simulink model "LMS_cs"  (R2023a)
settings: Solver=ode5  StartTime=0.0  StopTime=inf  FixedStep=1/200  RelTol=1e-3
PreLoadFcn:
  | mbxruntime.callbacks.PreLoadFcn(bdroot);
PostLoadFcn:
  | mbxruntime.callbacks.PostLoadFcn(bdroot);
InitFcn:
  | mbxruntime.callbacks.InitFcn(bdroot);
StartFcn:
  | mbxruntime.callbacks.StartFcn(bdroot);
StopFcn:
  | mbxruntime.callbacks.StopFcn(bdroot);
model workspace (MAT data in the model file):
  mbox_table : object (value not decoded)
  model_closed = 0
  sim_status = 0
undefined symbols (not defined in the file or in its folder): DiscIntNeverNeededParam, WheelL0, WheelL1, WheelR0, WheelR1
libraries: simulink x462, simulink_extras x117, PreScanSimulinkLibrary x33, PreScanUsefulBlocks x6, instrumentseriallib x5, simulink_need_slupdate x1
(part 7 of 68)

== system LMS_cs/WheelR1_BMW_X5_SUV_9 ==
  WheelR1_BMW_X5_SUV_9 : Inport  Tag=inport/JointActuator  OutDataTypeStr=Bus: PRESCAN_POSE_DATA  SampleTime=2/200  BusOutputAsStruct=on
  Actuator : Subsystem  Tag=VisuJoint  mask(PreScan Sink Block: VisuJoint){UniqueID=3670, Translate_ObjectID3D=BMW_X5_SUV_9.WheelR1, Rotate_ObjectID3D=BMW_X5_SUV_9.WheelR1, TimeStep=2/200, DisplayName=[]}
      mask prompts: UniqueID "Parent Unique ID"; Translate_ObjectID3D "Translate Object Name"; Rotate_ObjectID3D "Rotate Object Name"; TimeStep "Simulation Step"; DisplayName "Display Name"
      mask help:
      | The VisuJoint block provides a way to adapt the location and orientation of a part of an object.
      |
      | For more information, please click Help.
      settings: DeleteFcn=PreScanBlockDeleteFcn;
      mask Help: eval('openHelp(223)')
      mask Display: image(imread('Joint.png'))
  wires:
  WheelR1_BMW_X5_SUV_9/1 -> Actuator/1(Joint)

== system LMS_cs/Audi_A8_Sedan_1/BLR_Demux ==
  Radar : Inport
  Bus Selector1 : BusSelector  OutputSignals=ActiveBeamID[-],Range[m],DopplerVelocity[ms-1],DopplerVelocityX[ms-1],DopplerVelocityY[ms-1],DopplerVelocityZ[ms-1],Theta[deg],Phi[deg],TargetID[-],TargetTypeID[-],EnergyLoss[dB],Alpha[deg],Beta[deg]  OutputAsBus=on
  ScannerSensorLegacyBusConversion : PreScanUsefulBlocks/ScannerSensorLegacyBusConversion  MAXMESSAGES=MAXMESSAGES
  Radar Data : Outport
  wires:
  Bus Selector1/1 -> Radar Data/1
  ScannerSensorLegacyBusConversion/1 -> Bus Selector1/1
  Radar/1 -> ScannerSensorLegacyBusConversion/1

== system LMS_cs/Audi_A8_Sedan_1/BRR_Demux ==
  Radar : Inport
  Bus Selector1 : BusSelector  OutputSignals=ActiveBeamID[-],Range[m],DopplerVelocity[ms-1],DopplerVelocityX[ms-1],DopplerVelocityY[ms-1],DopplerVelocityZ[ms-1],Theta[deg],Phi[deg],TargetID[-],TargetTypeID[-],EnergyLoss[dB],Alpha[deg],Beta[deg]  OutputAsBus=on
  ScannerSensorLegacyBusConversion : PreScanUsefulBlocks/ScannerSensorLegacyBusConversion  MAXMESSAGES=MAXMESSAGES
  Radar Data : Outport
  wires:
  Bus Selector1/1 -> Radar Data/1
  ScannerSensorLegacyBusConversion/1 -> Bus Selector1/1
  Radar/1 -> ScannerSensorLegacyBusConversion/1

== system LMS_cs/Audi_A8_Sedan_1/Dynamics_Simple_3D ==
  DeltaSteer_[deg] : Inport
  Throttle : Inport  Port=2
  Brake : Inport  Port=3
  Initial_Vx_[ms-1] : Inport  Port=4
  AutoManual_OnOff : Inport  Port=5
  Auto_GearShift : Inport  Port=6
  Manual_GearShift : Inport  Port=7
  TyreInfo_in : Inport  Port=8
  Bus Creator : BusCreator  Inputs=14
  Bus Selector : BusSelector  OutputSignals=z_wheelFL_[m],z_wheelFR_[m],z_wheelRL_[m],z_wheelRR_[m]
  Chassis : Subsystem
      mask Display: image(imread('Chassis.png'));
  Engine : Subsystem
      mask Display: image(imread('Engine.png'));
  Gain : Gain  Gain=3.6
  Gear: Auto Manual : Subsystem
  Mux : Mux  Inputs=3
  Radians to Degrees : simulink_extras/Transformations/Radians to Degrees
  Radians to Degrees1 : simulink_extras/Transformations/Radians to Degrees
  Selector : Selector  InputPortWidth=9  IndexOptions=Index vector (dialog)  Indices=7  OutputSizes=1
  Selector1 : Selector  InputPortWidth=9  IndexOptions=Index vector (dialog)  Indices=8  OutputSizes=1
  ShiftLogic : Subsystem
      mask Display: image(imread('Gearshift.png'));
  Transmission : Subsystem
      mask Display: image(imread('Transmission.png'));
  State : Outport
  Vx [m s-1] : Outport  Port=2
  Perf_Params : Outport  Port=3
  z_wheelFL_[m] : Outport  Port=4
  z_wheelFR_[m] : Outport  Port=5
  z_wheelRL_[m] : Outport  Port=6
  z_wheelRR_[m] : Outport  Port=7
  ContactParams : Outport  Port=8
  wires:
  [ax] -> Bus Creator/4  "Ax_[ms-2]"
  [vx] -> Gain/1
  Selector1/1 -> Radians to Degrees1/1
  Selector/1 -> Radians to Degrees/1
  [PD] -> Bus Creator/10  "PDrive_[kW]"
  Radians to Degrees1/1 -> Bus Creator/12  "Pitch_[deg]"
  Radians to Degrees/1 -> Bus Creator/11  "Roll_[deg]"
  [PE] -> Bus Creator/9  "PEngine_[kW]"
  Bus Creator/1 -> Perf_Params/1
  Engine/2(PEngine_[kW]) -> [PE]
  [brake] -> Bus Creator/8  "Brake_[bar]"
  [throttle] -> Bus Creator/7  "Throttle_[perc]"
  [auto_manual] -> Bus Creator/6  "Auto_Manual_[-]"
  [ay] -> Bus Creator/5  "Ay_[ms-2]"
  [gear] -> Bus Creator/3  "Gear_[-]"
  [RPM] -> Bus Creator/2  "NEngine_[rpm]"
  Gain/1 -> Bus Creator/1  "Vx_[kmh-1]"
  Transmission/1(ImpellerTorque_[Nm]) -> Engine/1(ImpellerTorque_[Nm])  "ImpellerTorque_[Nm]"
  Transmission/2(TransmissionTorque_[Nm]) -> Chassis/1(TransmissionTorque_[Nm])  "TransmissionTorque_[Nm]"
  ShiftLogic/1(GearNr) -> ShiftLogic/2(GearNr_[-]), Gear: Auto Manual/3(Auto_Gear)  "GearNr_[-]"
  Engine/1(nEngine_[rpm]) -> Transmission/1(nEngine_[rpm]), [RPM]  "nEngine_[rpm]"
  Chassis/1(State) -> Selector1/1, Selector/1, State/1, Mux/1
  DeltaSteer_[deg]/1 -> Chassis/3(DeltaSteer_[deg])
  Initial_Vx_[ms-1]/1 -> Chassis/4(Initial_Vx_[ms-1])
  Throttle/1 -> [throttle], ShiftLogic/1(Throttle_[%]), Engine/2(Throttle_[%])
  Auto_GearShift/1 -> ShiftLogic/3(Auto_GearShift)
  Chassis/7(TransmissionOut_[rpm]) -> Transmission/3(n_TransmissionOut_[rpm])  "n_driveline_[rpm]"
  Chassis/2(VehicleSpeed_[ms-1]) -> [vx], Vx [m s-1]/1, Mux/2  "vx_[ms-1]"
  AutoManual_OnOff/1 -> [auto_manual], Gear: Auto Manual/1(Auto_Manual)
  Manual_GearShift/1 -> Gear: Auto Manual/2(Manual_Gear)
  Gear: Auto Manual/1(Gear) -> [gear], Transmission/2(GearNr_[-])  "gear"
  [vx] -> ShiftLogic/4(VehSpeed_[ms-1])
  TyreInfo_in/1 -> Chassis/5(TyreInfo_in)
  Brake/1 -> Chassis/2(BrakePressure_[bar]), [brake]
  Chassis/6(PDrive_[kW]) -> [PD]
  Chassis/5(ay_[ms-2]) -> [ay]
  Chassis/4(ax_[ms-2]) -> [ax]
  Chassis/3(Vy_[ms-1]) -> [vy]
  [vx] -> Bus Creator/13  "vx_[ms-1]"
  [vy] -> Bus Creator/14  "vy_[ms-1]"
  Chassis/8(z_wheel_[m]) -> Bus Selector/1, Mux/3  "z_wheel_[m]"
  Bus Selector/1 -> z_wheelFL_[m]/1  "<z_wheelFL_[m]>"
  Bus Selector/2 -> z_wheelFR_[m]/1  "<z_wheelFR_[m]>"
  Bus Selector/3 -> z_wheelRL_[m]/1  "<z_wheelRL_[m]>"
  Bus Selector/4 -> z_wheelRR_[m]/1  "<z_wheelRR_[m]>"
  Mux/1 -> ContactParams/1

== system LMS_cs/Audi_A8_Sedan_1/FLR_Demux ==
  Radar : Inport
  Bus Selector1 : BusSelector  OutputSignals=ActiveBeamID[-],Range[m],DopplerVelocity[ms-1],DopplerVelocityX[ms-1],DopplerVelocityY[ms-1],DopplerVelocityZ[ms-1],Theta[deg],Phi[deg],TargetID[-],TargetTypeID[-],EnergyLoss[dB],Alpha[deg],Beta[deg]  OutputAsBus=on
  ScannerSensorLegacyBusConversion : PreScanUsefulBlocks/ScannerSensorLegacyBusConversion  MAXMESSAGES=MAXMESSAGES
  Radar Data : Outport
  wires:
  Bus Selector1/1 -> Radar Data/1
  ScannerSensorLegacyBusConversion/1 -> Bus Selector1/1
  Radar/1 -> ScannerSensorLegacyBusConversion/1

== system LMS_cs/Audi_A8_Sedan_1/FRR_Demux ==
  Radar : Inport
  Bus Selector1 : BusSelector  OutputSignals=ActiveBeamID[-],Range[m],DopplerVelocity[ms-1],DopplerVelocityX[ms-1],DopplerVelocityY[ms-1],DopplerVelocityZ[ms-1],Theta[deg],Phi[deg],TargetID[-],TargetTypeID[-],EnergyLoss[dB],Alpha[deg],Beta[deg]  OutputAsBus=on
  ScannerSensorLegacyBusConversion : PreScanUsefulBlocks/ScannerSensorLegacyBusConversion  MAXMESSAGES=MAXMESSAGES
  Radar Data : Outport
  wires:
  Bus Selector1/1 -> Radar Data/1
  ScannerSensorLegacyBusConversion/1 -> Bus Selector1/1
  Radar/1 -> ScannerSensorLegacyBusConversion/1

== system LMS_cs/Audi_A8_Sedan_1/JointGroup_WheelDisplacement_V2R ==
  Velocity [m/s] : Inport  SampleTime=TimeStep
  Discrete-Time Integrator : DiscreteIntegrator  SampleTime=TimeStep  ICPrevOutput=DiscIntNeverNeededParam  ICPrevScaledInput=DiscIntNeverNeededParam
  omega=V/Rwheel : Gain  Gain=1/TireRadius
  Rotation [rad] : Outport
  wires:
  Discrete-Time Integrator/1 -> Rotation [rad]/1  "roty"
  omega=V/Rwheel/1 -> Discrete-Time Integrator/1  "rotational speed [rad/s]"
  Velocity [m/s]/1 -> omega=V/Rwheel/1

== system LMS_cs/Audi_A8_Sedan_1/LRR_Demux ==
  Radar : Inport
  Bus Selector1 : BusSelector  OutputSignals=ActiveBeamID[-],Range[m],DopplerVelocity[ms-1],DopplerVelocityX[ms-1],DopplerVelocityY[ms-1],DopplerVelocityZ[ms-1],Theta[deg],Phi[deg],TargetID[-],TargetTypeID[-],EnergyLoss[dB],Alpha[deg],Beta[deg]  OutputAsBus=on
  ScannerSensorLegacyBusConversion : PreScanUsefulBlocks/ScannerSensorLegacyBusConversion  MAXMESSAGES=MAXMESSAGES
  Radar Data : Outport
  wires:
  Bus Selector1/1 -> Radar Data/1
  ScannerSensorLegacyBusConversion/1 -> Bus Selector1/1
  Radar/1 -> ScannerSensorLegacyBusConversion/1

== system LMS_cs/Audi_A8_Sedan_1/Lane Keeping Algorithm ==
  Sensor Data : Inport
  Add : Sum
  Add1 : Sum
  Add2 : Sum
  Bus Selector : BusSelector  OutputSignals=ScanAtSensor.SliceCenterCoordsX,ScanAtSensor.SliceCenterCoordsY,ScanAtDistance1.SliceCenterCoordsX,ScanAtDistance1.SliceCenterCoordsY,ScanAtSensor.RightLaneIntersection1.WorldCoordinateX,ScanAtSensor.RightLaneIntersection1.WorldCoordinateY,ScanAtDistance1.RightLaneIntersection1.WorldCoordinateX,ScanAtDistance1.RightLaneIntersection1.WorldCoordinateY
  Bus Selector1 : BusSelector  OutputSignals=ScanAtDistance1.LeftLaneIntersection1.DistanceFromScanCenter,ScanAtDistance1.RightLaneIntersection1.DistanceFromScanCenter,ScanAtDistance1.RoadIdUnderSliceCenter
  Constant : Constant  Value=-0.5
  Display{,1..18} (19 alike) : Display
  Divide : Product  Inputs=/*
  Scaler1 : Constant  Value=1250
  Scaler2 : Gain  Gain=-250
  Steering 0 : Constant  Value=0
  Switch : Switch  Criteria=u2 > Threshold  SaturateOnIntegerOverflow=off  InputSameDT=off
  "angular error " : M-S-Function  FunctionName=angular_error_msfun
      mask Display:
      | port_label('input',1,'cx1')
      | port_label('input',2,'cy1')
      | port_label('input',3,'cx2')
      | port_label('input',4,'cy2')
      | port_label('input',5,'lsx1')
      | port_label('input',6,'lsy1')
      | port_label('input',7,'lsx2')
      | port_label('input',8,'lsy2')
      | port_label('input',9,'scaler')
      | port_label('output',1,'angle')
  Steering Angle : Outport
  wires:
  Switch/1 -> Steering Angle/1
  Steering 0/1 -> Switch/3
  Bus Selector1/3 -> Display2/1, Switch/2  "<RoadIdUnderSliceCenter>"
  Add2/1 -> Display1/1, Switch/1
  Sensor Data/1 -> Bus Selector1/1, Bus Selector/1
  Bus Selector1/1 -> Display12/1, Display4/1, Add/1  "<DistanceFromScanCenter>"
  Bus Selector1/2 -> Display13/1, Divide/2, Add/2  "<DistanceFromScanCenter>"
  Add/1 -> Display14/1, Divide/1
  Divide/1 -> Display16/1, Display15/1, Add1/2
  Constant/1 -> Add1/1
  Add1/1 -> Display17/1, Scaler2/1
  Scaler2/1 -> Display18/1, Add2/2
  Bus Selector/1 -> Display3/1, "angular error "/1  "<SliceCenterCoordsX>"
  Bus Selector/2 -> Display5/1, "angular error "/2  "<SliceCenterCoordsY>"
  Bus Selector/3 -> Display6/1, "angular error "/3  "<SliceCenterCoordsX>"
  Bus Selector/4 -> "angular error "/4, Display7/1  "<SliceCenterCoordsY>"
  Bus Selector/5 -> Display8/1, "angular error "/5  "<WorldCoordinateX>"
  Bus Selector/6 -> Display9/1, "angular error "/6  "<WorldCoordinateY>"
  Bus Selector/7 -> Display10/1, "angular error "/7  "<WorldCoordinateX>"
  Bus Selector/8 -> Display11/1, "angular error "/8  "<WorldCoordinateY>"
  "angular error "/1 -> Display/1, Add2/1
  Scaler1/1 -> "angular error "/9

== system LMS_cs/Audi_A8_Sedan_1/LaneMarkerSensor_1_Data ==
  In1 : Inport
  Bus Creator : BusCreator  Inputs='SliceCount','ScanAtSensor','ScanAtDistance1','ScanAtDistance2','ScanAtDistance3'
  Constant : Constant
  Constant1 : Constant  Value=NUMBEROFSLICES
  Constant2 : Constant  Value=2
  Constant3 : Constant  Value=3
  Constant4 : Constant  Value=4
  Data Type Conversion : DataTypeConversion  OutDataTypeStr=int32  SaturateOnIntegerOverflow=off  RndMeth=Floor
  If{,1..3} (4 alike) : If  NumInputs=2  IfExpression=u1 >= u2  ShowElse=off
  If Action Subsystem1 : Subsystem  TreatAsAtomicUnit=on
  If Action Subsystem2 : Subsystem  TreatAsAtomicUnit=on
  If Action Subsystem3 : Subsystem  TreatAsAtomicUnit=on
  If Action Subsystem4 : Subsystem  TreatAsAtomicUnit=on
  Merge{,1..3} (4 alike) : Merge  InitialOutput=0
  Zero-filled data bus{,1..3} (4 alike) : Constant  Value=0  VectorParams1D=off  OutDataTypeStr=Bus: PRESCAN_LANEMARKER_DATA  SampleTime=TimeStep
  Detection Data : Outport
  wires:
  Data Type Conversion/1 -> Bus Creator/1  "SliceCount"
  In1/1 -> If Action Subsystem2/1(In1), If Action Subsystem4/1(In1), If Action Subsystem3/1(In1), If Action Subsystem1/1(In1)
  Zero-filled data bus3/1 -> Merge3/1
  Zero-filled data bus2/1 -> Merge2/1
  Zero-filled data bus1/1 -> Merge1/1
  Zero-filled data bus/1 -> Merge/1
  Merge3/1 -> Bus Creator/5  "ScanAtDistance3"
  Merge2/1 -> Bus Creator/4  "ScanAtDistance2"
  Merge1/1 -> Bus Creator/3  "ScanAtDistance1"
  If3/1 -> If Action Subsystem4/Action
  If Action Subsystem4/1(Out1) -> Merge3/2
  Constant4/1 -> If3/2, If Action Subsystem4/2(In2)
  If2/1 -> If Action Subsystem3/Action
  If Action Subsystem3/1(Out1) -> Merge2/2
  Constant3/1 -> If Action Subsystem3/2(In2), If2/2
  If1/1 -> If Action Subsystem1/Action
  If Action Subsystem1/1(Out1) -> Merge1/2
  Constant2/1 -> If Action Subsystem1/2(In2), If1/2
  Merge/1 -> Bus Creator/2  "ScanAtSensor"
  Bus Creator/1 -> Detection Data/1
  If/1 -> If Action Subsystem2/Action
  If Action Subsystem2/1(Out1) -> Merge/2
  Constant/1 -> If Action Subsystem2/2(In2), If/2
  Constant1/1 -> Data Type Conversion/1, If3/1, If2/1, If1/1, If/1

== system LMS_cs/Audi_A8_Sedan_1/PathFollower_1 ==
  TrajOffset_x,y,Y [m,m,deg] : Inport
  ActorOffset_Left(+) / Right(-) [m] : Inport  Port=2
  position x,y,Y [m,m,deg] : Inport  Port=3
  Initial Velocity [m/s] : Inport  Port=4
  Desired Velocity [m/s] : Inport  Port=5
  velocity [m/s] : Inport  Port=6
  CTRL REFERENCES : Subsystem
  Calculate shifted p0 wrt COG : Subsystem
  DELTA CTRL : Subsystem
  Demux : Demux  Outputs=3
  Gain : Gain  Gain=1*pi/180
  Goto Tag Visibility : GotoTagVisibility  GotoTag=PreviewDistance
  Goto Tag Visibility1 : GotoTagVisibility  GotoTag=v_actual
  Memory1 : Memory
  Memory2 : Memory
  Memory3 : Memory
  Mux : Mux  Inputs=3
  Preview distance velocity dependent : Lookup  InputValues=[0 20 30 40 50 60 70 80 90 100 120]  Table=[1 1 2 3 4 5 6 7 10 13.33 20]  SaturateOnIntegerOverflow=off
  THROTTLE CTRL : Subsystem
  sign1 : Gain  Gain=3.6
  delta_steerwheel [deg] : Outport
  throttle [%] : Outport  Port=2
  brake pressure [bar] : Outport  Port=3
  v0 [m/s] : Outport  Port=4
  Auto_GearShift : Outport  Port=5
  Actor/Traj_distance [m] : Outport  Port=6
  Actor/Traj_angle [deg] : Outport  Port=7
  tag scope: PreviewDistance=scoped, v_actual=scoped
  wires:
  Memory3/1 -> CTRL REFERENCES/4(ActorOffset_Left(+) / Right(-)_[m])
  THROTTLE CTRL/4(Auto_GearShift) -> Auto_GearShift/1
  THROTTLE CTRL/2(brake pressure [bar]) -> brake pressure [bar]/1
  Memory2/1 -> THROTTLE CTRL/1(v_actual [m/s]), [v_actual]
  Memory1/1 -> DELTA CTRL/1(p0), CTRL REFERENCES/1(Pos x,y,Y [m,m,rad])
  sign1/1 -> Preview distance velocity dependent/1
  Initial Velocity [m/s]/1 -> THROTTLE CTRL/3(Initial Velocity [m/s])
  velocity [m/s]/1 -> Memory2/1
  CTRL REFERENCES/1(pvp  [m,m]) -> DELTA CTRL/2(pvp)
  CTRL REFERENCES/2(pref_pvp [m,m]) -> DELTA CTRL/3(pref_pvp)
  Gain/1 -> Mux/3
  DELTA CTRL/1(delta_steerwheel [deg]) -> delta_steerwheel [deg]/1
  Mux/1 -> CTRL REFERENCES/3(TrajOffset [m,m,rad])
  CTRL REFERENCES/3(pref_0 [m,m]) -> DELTA CTRL/4(pref0)
  THROTTLE CTRL/3(v0 [m/s]) -> v0 [m/s]/1
  THROTTLE CTRL/1(throttle [%]) -> throttle [%]/1
  [v_actual] -> sign1/1
  Preview distance velocity dependent/1 -> [PreviewDistance], CTRL REFERENCES/2(Position Preview Distance [m])
  Desired Velocity [m/s]/1 -> THROTTLE CTRL/2(Desired Velocity [m/s])
  ActorOffset_Left(+) / Right(-) [m]/1 -> Memory3/1
  Demux/1 -> Mux/1
  Demux/2 -> Mux/2
  Demux/3 -> Gain/1
  TrajOffset_x,y,Y [m,m,deg]/1 -> Demux/1
  Calculate shifted p0 wrt COG/1(position x,y,Y [m,m,rad]) -> Memory1/1
  position x,y,Y [m,m,deg]/1 -> Calculate shifted p0 wrt COG/1(position x,y,Y [m,m,deg])
  CTRL REFERENCES/4(Actor/Traj_distance [m]) -> Actor/Traj_distance [m]/1
  CTRL REFERENCES/5(Actor/Traj_angle [deg]) -> Actor/Traj_angle [deg]/1

== system LMS_cs/Audi_A8_Sedan_1/PreScan_Contact_Sensor ==
  ContactParams : Inport  SampleTime=TimeStep
  Steer Angle Front [deg] : Inport  Port=2
  Steer Angle Rear [deg] : Inport  Port=3
  Bus Creator2 : BusCreator  Inputs=4
  Demux : Demux
  Demux1 : Demux  Outputs=[9 1 4]
  Demux2 : Demux
  For All Wheel Contacts : Subsystem  TreatAsAtomicUnit=on
  Mux6 : Mux  Inputs=2
  Subsystem : Subsystem  mask{NumberOfWheels=4, MaxContactPoints=4, WheelRadius=wheelRadius, WheelWidth=0.2}
      mask prompts: NumberOfWheels "Number of Wheels"; MaxContactPoints "Maximum number of Contact Points"; WheelRadius "Wheel Radius"; WheelWidth "Wheel Width"
      mask Display: disp('Contact Sensor')
  Tire Collision Demux : Subsystem
  Tire Collision Demux1 : Subsystem
  Tire Collision Demux2 : Subsystem
  Tire Collision Demux3 : Subsystem
  Vehicle Local to World : Subsystem
  Wheels = 4 : Subsystem  mask{NumberOfWheels=4}
      mask prompts: NumberOfWheels "Number of Wheels"
      mask Display:
      | port_label('input', 1,'Vehicle wrt World')
      | port_label('input', 2,'Wheels wrt World')
  Wheels Local to World : Subsystem  Tag=MuxWheels  mask(PreScan Mux Block:){}
      settings: DeleteFcn=PreScanBlockDeleteFcn;
  Results : Outport
  wires:
  Mux6/1 -> Wheels = 4/1(Vehicle wrt World)
  Wheels = 4/1(WheelPoses) -> Subsystem/1(In1)
  Demux/1 -> Tire Collision Demux/1(demux in)
  Demux/2 -> Tire Collision Demux1/1(demux in)
  Demux/3 -> Tire Collision Demux2/1(demux in)
  Demux/4 -> Tire Collision Demux3/1(demux in)
  Tire Collision Demux/1(bus out) -> Bus Creator2/1  "TireFL"
  Tire Collision Demux1/1(bus out) -> Bus Creator2/2  "TireFR"
  Tire Collision Demux2/1(bus out) -> Bus Creator2/3  "TireRL"
  Tire Collision Demux3/1(bus out) -> Bus Creator2/4  "TireRR"
  Vehicle Local to World/1(Position) -> Mux6/1
  Vehicle Local to World/2(Orientation) -> Mux6/2
  Wheels Local to World/1(Wheel Poses) -> Wheels = 4/2(Wheels wrt World)
  Demux1/2 -> Wheels Local to World/3(Velocity [m/s])
  Demux2/1 -> Wheels Local to World/4(zDisp FL [m])
  Demux2/2 -> Wheels Local to World/5(zDisp FR [m])
  Demux2/3 -> Wheels Local to World/6(zDisp RL [m])
  Demux2/4 -> Wheels Local to World/7(zDisp RR [m])
  Steer Angle Front [deg]/1 -> Wheels Local to World/1(Steer Angle Front [deg])
  Steer Angle Rear [deg]/1 -> Wheels Local to World/2(Steer Angle Rear [deg])
  Bus Creator2/1 -> Results/1
  ContactParams/1 -> Demux1/1
  Demux1/1 -> Vehicle Local to World/1(State)
  Demux1/3 -> Demux2/1
  Subsystem/1(Out1) -> For All Wheel Contacts/1(In1)
  For All Wheel Contacts/1(Out1) -> Demux/1

== system LMS_cs/Audi_A8_Sedan_1/SELF_Demux ==
  SELF : Inport  OutDataTypeStr=Bus: PRESCAN_SELFSENSORDATA
  Bus Selector : BusSelector  OutputSignals=PositionX,PositionY,PositionZ,OrientationRoll,OrientationPitch,OrientationYaw,Velocity,Yaw_rate,Lat,Long,Alt
  Demux2 : Demux  Outputs=3
  Gain : Gain  Gain=180/pi
  Gain1 : Gain  Gain=180/pi
  Vector Concatenate1 : Concatenate  NumInputs=3
  compas converter : Subsystem
  x [m] : Outport
  y [m] : Outport  Port=2
  z [m] : Outport  Port=3
  rotx [deg] : Outport  Port=4
  roty [deg] : Outport  Port=5
  rotz [deg] : Outport  Port=6
  GPS lat [deg] : Outport  Port=7
  GPS long [deg] : Outport  Port=8
  GPS alt [m] : Outport  Port=9
  velocity [m/s] : Outport  Port=10
  heading [deg] : Outport  Port=11
  yaw rate [deg/s] : Outport  Port=12
  wires:
  Bus Selector/11 -> GPS alt [m]/1  "<Alt>"
  Bus Selector/10 -> GPS long [deg]/1  "<Long>"
  Bus Selector/9 -> GPS lat [deg]/1  "<Lat>"
  Bus Selector/8 -> Gain1/1  "<Yaw_rate>"
  Bus Selector/7 -> velocity [m/s]/1  "<Velocity>"
  Bus Selector/6 -> compas converter/1(rotz [rad]), Vector Concatenate1/3  "<OrientationYaw>"
  Bus Selector/5 -> Vector Concatenate1/2  "<OrientationPitch>"
  Bus Selector/4 -> Vector Concatenate1/1  "<OrientationRoll>"
  Vector Concatenate1/1 -> Gain/1
  Bus Selector/3 -> z [m]/1  "<PositionZ>"
  Bus Selector/2 -> y [m]/1  "<PositionY>"
  Bus Selector/1 -> x [m]/1  "<PositionX>"
  SELF/1 -> Bus Selector/1
  Gain/1 -> Demux2/1
  Demux2/1 -> rotx [deg]/1
  Demux2/2 -> roty [deg]/1
  Demux2/3 -> rotz [deg]/1
  compas converter/1(heading [deg]) -> heading [deg]/1
  Gain1/1 -> yaw rate [deg/s]/1

== system LMS_cs/Audi_A8_Sedan_1/SRR_Demux ==
  Radar : Inport
  Bus Selector1 : BusSelector  OutputSignals=ActiveBeamID[-],Range[m],DopplerVelocity[ms-1],DopplerVelocityX[ms-1],DopplerVelocityY[ms-1],DopplerVelocityZ[ms-1],Theta[deg],Phi[deg],TargetID[-],TargetTypeID[-],EnergyLoss[dB],Alpha[deg],Beta[deg]  OutputAsBus=on
  ScannerSensorLegacyBusConversion : PreScanUsefulBlocks/ScannerSensorLegacyBusConversion  MAXMESSAGES=MAXMESSAGES
  Radar Data : Outport
  wires:
  Bus Selector1/1 -> Radar Data/1
  ScannerSensorLegacyBusConversion/1 -> Bus Selector1/1
  Radar/1 -> ScannerSensorLegacyBusConversion/1

== system LMS_cs/Audi_A8_Sedan_1/STATE_Audi_A8_Sedan_1 ==
  State : Inport  SampleTime=TimeStep
  Bus Creator : BusCreator  Inputs=15  OutDataTypeStr=Bus: PRESCAN_STATEACTUATORDATA  NonVirtualBus=on
  Demux : Demux  Outputs=15
  iniBODYAngles wrtVEH [rad] : Constant  Value=[Roll0 Pitch0 0]  SampleTime=TimeStep
  iniVEHAngles wrtGLOB [rad] : Constant  Value=[0 0 Yaw0]  SampleTime=TimeStep
  iniVEHposition wrtGLOB [m] : Constant  Value=[x0 y0 z0]  SampleTime=TimeStep
  state2FullState : PreScanSimulinkLibrary/state2FullState  SystemSampleTime=-1  VariantActivationTime=update diagram  Latency=0  AutoFrameSizeCalculation=off
  StateBus : Outport  OutDataTypeStr=Bus: PRESCAN_STATEACTUATORDATA
  wires:
  Bus Creator/1 -> StateBus/1
  State/1 -> state2FullState/1
  state2FullState/1 -> Demux/1
  iniVEHposition wrtGLOB [m]/1 -> state2FullState/2
  iniBODYAngles wrtVEH [rad]/1 -> state2FullState/3
  iniVEHAngles wrtGLOB [rad]/1 -> state2FullState/4
  Demux/1 -> Bus Creator/1  "PositionX"
  Demux/2 -> Bus Creator/2  "PositionY"
  Demux/3 -> Bus Creator/3  "PositionZ"
  Demux/4 -> Bus Creator/4  "VelocityX"
  Demux/5 -> Bus Creator/5  "VelocityY"
  Demux/6 -> Bus Creator/6  "VelocityZ"
  Demux/7 -> Bus Creator/7  "AccelerationX"
  Demux/8 -> Bus Creator/8  "AccelerationY"
  Demux/9 -> Bus Creator/9  "AccelerationZ"
  Demux/10 -> Bus Creator/10  "OrientationRoll"
  Demux/11 -> Bus Creator/11  "OrientationPitch"
  Demux/12 -> Bus Creator/12  "OrientationYaw"
  Demux/13 -> Bus Creator/13  "AngularVelocityRoll"
  Demux/14 -> Bus Creator/14  "AngularVelocityPitch"
  Demux/15 -> Bus Creator/15  "AngularVelocityYaw"

== system LMS_cs/Audi_A8_Sedan_1/State2PathFollowerCnv ==
  State BUS : Inport  OutDataTypeStr=Bus: PRESCAN_STATEACTUATORDATA
  Bus Selector : BusSelector  OutputSignals=AngularVelocityYaw,VelocityX,VelocityY,PositionX,PositionY,OrientationYaw
  Radians to Degrees : simulink_extras/Transformations/Radians to Degrees
  Radians to Degrees1 : simulink_extras/Transformations/Radians to Degrees
  SELF2PathFollowerMux : Mux  Tag=SELF2PathFollowerMux  Inputs=3
  velocity magnitude : Math  Operator=hypot  SignedPower=on
  Yaw rate [deg/s] : Outport
  velocity [m/s] : Outport  Port=2
  position x,y,Y [m,m,deg] : Outport  Port=3
  wires:
  Radians to Degrees1/1 -> Yaw rate [deg/s]/1
  Bus Selector/1 -> Radians to Degrees1/1  "<AngularVelocityYaw>"
  velocity magnitude/1 -> velocity [m/s]/1
  SELF2PathFollowerMux/1 -> position x,y,Y [m,m,deg]/1
  State BUS/1 -> Bus Selector/1
  Bus Selector/2 -> velocity magnitude/1  "<VelocityX>"
  Bus Selector/3 -> velocity magnitude/2  "<VelocityY>"
  Radians to Degrees/1 -> SELF2PathFollowerMux/3
  Bus Selector/6 -> Radians to Degrees/1  "<OrientationYaw>"
  Bus Selector/4 -> SELF2PathFollowerMux/1  "<PositionX>"
  Bus Selector/5 -> SELF2PathFollowerMux/2  "<PositionY>"

== system LMS_cs/Audi_A8_Sedan_1/Trajectories ==
  Traj2State1 : Subsystem  Tag=Traj2State  mask(PreScan Demux Block:){}
      settings: DeleteFcn=PreScanBlockDeleteFcn;
  TrajCoGOffset : Subsystem  Tag=TrajCoGOffset  mask(Trajectory CoG Offset block){CoGOffsetZ=0.55, InitRoll=0, InitPitch=0}
      mask prompts: CoGOffsetZ "Z-component of CoG Offset [m]:"; InitRoll "Initial Roll angle [deg]:"; InitPitch "Initial Pitch angle [deg]:"
      mask help: A trajectory follows the surface of the road. However the position of a actor is based on the actor's Center of Gravity, which is typically above the road. This block converts from the trajectory along the road surface to the trajectory of the actor's CoG by realigning the z-component of the CoG offset to be normal to the road.
      settings: DeleteFcn=PreScanBlockDeleteFcn;
  Trajectory_1 : Subsystem  Tag=Trajectory  mask(PreScan Source Block: Trajectory){FileName='Trajectory_1.mat', TimeStep=2/200}
      mask prompts: TimeStep "Time Step [s]"
      mask help:
      | The Trajectory block contains the trajectories defined in the PreScan Experiment Editor. The output of the trajectory block is the (vehicle) State.
      |
      | For more information, please click Help.
      mask init:
      | EXPROOT=pwd;  % TODO better construction for locating base experiment
      | 
      | trajfilename = fullfile(EXPROOT,'Trajectories',FileName);
      | load(trajfilename);
      | trajectory=trajectory';
      | 
      | traj.time=trajectory(:,1);%[];
      | traj.signals.values=trajectory(:,2:19);
      | traj.dimensions=18;
      | traj.label='';
      | 
      | SampleTime=traj.time(2)-traj.time(1);
      settings: DeleteFcn=PreScanBlockDeleteFcn;
      mask Help: eval('openHelp(312)')
      mask Display: fprintf(FileName)
  Trajectory_1_Offset : Constant  Tag=TrajectoryOffset  Value="[0  0  0  0  0  0]"
  State : Outport  Tag=TrajOutport
  wires:
  Trajectory_1/1(trajectory) -> Traj2State1/1(Traj Org)
  Trajectory_1_Offset/1 -> Traj2State1/2(Offset)
  TrajCoGOffset/1(State Out) -> State/1
  Traj2State1/1(state) -> TrajCoGOffset/1(State In)

== system LMS_cs/Audi_A8_Sedan_1/WheelDisplacement_Mux ==
  Steering Angle Front [rad] : Inport  Tag=inport/JointGroup  SampleTime=2/200  BusOutputAsStruct=on
  Steering Angle Rear [rad] : Inport  Tag=inport/JointGroup  Port=2  SampleTime=2/200  BusOutputAsStruct=on
  Rotation [rad] : Inport  Tag=inport/JointGroup  Port=3  SampleTime=2/200  BusOutputAsStruct=on
  zDisp FL [m] : Inport  Tag=inport/JointGroup  Port=4  SampleTime=2/200  BusOutputAsStruct=on
  zDisp FR [m] : Inport  Tag=inport/JointGroup  Port=5  SampleTime=2/200  BusOutputAsStruct=on
  zDisp RL [m] : Inport  Tag=inport/JointGroup  Port=6  SampleTime=2/200  BusOutputAsStruct=on
  zDisp RR [m] : Inport  Tag=inport/JointGroup  Port=7  SampleTime=2/200  BusOutputAsStruct=on
  Ground_{1..12} (12 alike) : Ground
  WheelL0_Mux : Subsystem  Tag=mux/Joint  mask(PreScan Mux Block){DisplayName=WheelL0}
      mask prompts: DisplayName "Display Name"
      mask help:
      | This block simulates a generic joint used for generic models. This joint can be enabled/disabled from the GUI.
      |
      | For more information, please click Help.
      settings: DeleteFcn=PreScanBlockDeleteFcn;
      mask Help: eval('openHelp(254)')
  WheelL1_Mux : Subsystem  Tag=mux/Joint  mask(PreScan Mux Block){DisplayName=WheelL1}
      mask prompts: DisplayName "Display Name"
      mask help:
      | This block simulates a generic joint used for generic models. This joint can be enabled/disabled from the GUI.
      |
      | For more information, please click Help.
      settings: DeleteFcn=PreScanBlockDeleteFcn;
      mask Help: eval('openHelp(254)')
  WheelR0_Mux : Subsystem  Tag=mux/Joint  mask(PreScan Mux Block){DisplayName=WheelR0}
      mask prompts: DisplayName "Display Name"
      mask help:
      | This block simulates a generic joint used for generic models. This joint can be enabled/disabled from the GUI.
      |
      | For more information, please click Help.
      settings: DeleteFcn=PreScanBlockDeleteFcn;
      mask Help: eval('openHelp(254)')
  WheelR1_Mux : Subsystem  Tag=mux/Joint  mask(PreScan Mux Block){DisplayName=WheelR1}
      mask prompts: DisplayName "Display Name"
      mask help:
      | This block simulates a generic joint used for generic models. This joint can be enabled/disabled from the GUI.
      |
      | For more information, please click Help.
      settings: DeleteFcn=PreScanBlockDeleteFcn;
      mask Help: eval('openHelp(254)')
  WheelL0_Audi_A8_Sedan_1 : Outport  Tag=outport/JointActuator  OutDataTypeStr=Bus: PRESCAN_POSE_DATA  SampleTime=2/200
  WheelL1_Audi_A8_Sedan_1 : Outport  Tag=outport/JointActuator  Port=2  OutDataTypeStr=Bus: PRESCAN_POSE_DATA  SampleTime=2/200
  WheelR0_Audi_A8_Sedan_1 : Outport  Tag=outport/JointActuator  Port=3  OutDataTypeStr=Bus: PRESCAN_POSE_DATA  SampleTime=2/200
  WheelR1_Audi_A8_Sedan_1 : Outport  Tag=outport/JointActuator  Port=4  OutDataTypeStr=Bus: PRESCAN_POSE_DATA  SampleTime=2/200
  wires:
  WheelL0_Mux/1(Joint) -> WheelL0_Audi_A8_Sedan_1/1
  WheelL1_Mux/1(Joint) -> WheelL1_Audi_A8_Sedan_1/1
  WheelR0_Mux/1(Joint) -> WheelR0_Audi_A8_Sedan_1/1
  WheelR1_Mux/1(Joint) -> WheelR1_Audi_A8_Sedan_1/1
  Steering Angle Front [rad]/1 -> WheelR0_Mux/6(Yaw [rad]), WheelL0_Mux/6(Yaw [rad])
  Steering Angle Rear [rad]/1 -> WheelR1_Mux/6(Yaw [rad]), WheelL1_Mux/6(Yaw [rad])
  Rotation [rad]/1 -> WheelR0_Mux/5(Pitch [rad]), WheelL0_Mux/5(Pitch [rad]), WheelR1_Mux/5(Pitch [rad]), WheelL1_Mux/5(Pitch [rad])
  zDisp FL [m]/1 -> WheelL0_Mux/3(Z [m])
  zDisp FR [m]/1 -> WheelR0_Mux/3(Z [m])
  zDisp RL [m]/1 -> WheelL1_Mux/3(Z [m])
  zDisp RR [m]/1 -> WheelR1_Mux/3(Z [m])
  Ground_1/1 -> WheelL0_Mux/1(X [m])
  Ground_2/1 -> WheelL0_Mux/2(Y [m])
  Ground_3/1 -> WheelL0_Mux/4(Roll [rad])
  Ground_4/1 -> WheelL1_Mux/1(X [m])
  Ground_5/1 -> WheelL1_Mux/2(Y [m])
  Ground_6/1 -> WheelL1_Mux/4(Roll [rad])
  Ground_7/1 -> WheelR0_Mux/1(X [m])
  Ground_8/1 -> WheelR0_Mux/2(Y [m])
  Ground_9/1 -> WheelR0_Mux/4(Roll [rad])
  Ground_10/1 -> WheelR1_Mux/1(X [m])
  Ground_11/1 -> WheelR1_Mux/2(Y [m])
  Ground_12/1 -> WheelR1_Mux/4(Roll [rad])

== system LMS_cs/Audi_A8_Sedan_1/concatinate Frame ==
  " Desired Velocity" : Inport
  Heading : Inport  Port=2
  " LRR_Range" : Inport  Port=3
  LRR_RelativeVelocity : Inport  Port=4
  " SRR_Range" : Inport  Port=5
  " SRR_RelativeVelocity" : Inport  Port=6
  " FLR_Range" : Inport  Port=7
  " FLR_RelativeVelocity" : Inport  Port=8
  FLR_Azimuth : Inport  Port=9
  " FRR_Range" : Inport  Port=10
  " FRR_RelativeVelocity" : Inport  Port=11
  " FRR_Azimuth" : Inport  Port=12
  " BRR_Range" : Inport  Port=13
  " BRR_RelativeVelocity" : Inport  Port=14
  " BRR_Azimuth" : Inport  Port=15
  " BLR_Range" : Inport  Port=16
  " BLR_RelativeVelocity" : Inport  Port=17
  " BLR_Azimuth" : Inport  Port=18
  Velocity : Inport  Port=19
  laneMarkerX_D0 : Inport  Port=20
  laneMarkerY_D0 : Inport  Port=21
  laneMarkerX_D1 : Inport  Port=22
  laneMarkerY_D1 : Inport  Port=23
  worldrX_D0 : Inport  Port=24
  worldY_D0 : Inport  Port=25
  worldX_D1 : Inport  Port=26
  worldY_D1 : Inport  Port=27
  laneMarkerLeft_D1 : Inport  Port=28
  laneMarkerRight_D1 : Inport  Port=29
  roadID : Inport  Port=30
  String Concatenate : StringConcatenate  Inputs=61
  String Constant : StringConstant  String="\"*\""
  String Constant{1..4,6..30} (29 alike) : StringConstant  String="\";\""
  String Constant5 : StringConstant  String="\"#\""
  String to ASCII : StringToASCII  OutputVectorSize=255
  To String{,1..29} (30 alike) : ToString
  Frame : Outport  VectorParamsAs1DForOutWhenUnconnected=off
  wires:
  String to ASCII/1 -> Frame/1
  " SRR_Range"/1 -> To String4/1
  To String4/1 -> String Concatenate/10
  String Constant3/1 -> String Concatenate/7
  Heading/1 -> To String1/1
  To String2/1 -> String Concatenate/6
  String Constant1/1 -> String Concatenate/3
  " Desired Velocity"/1 -> To String/1
  String Constant/1 -> String Concatenate/1
  " LRR_Range"/1 -> To String2/1
  To String1/1 -> String Concatenate/4
  To String3/1 -> String Concatenate/8
  To String/1 -> String Concatenate/2
  LRR_RelativeVelocity/1 -> To String3/1
  String Constant4/1 -> String Concatenate/9
  String Constant2/1 -> String Concatenate/5
  String Concatenate/1 -> String to ASCII/1
  String Constant6/1 -> String Concatenate/11
  String Constant7/1 -> String Concatenate/13
  String Constant8/1 -> String Concatenate/15
  String Constant9/1 -> String Concatenate/17
  String Constant10/1 -> String Concatenate/19
  String Constant11/1 -> String Concatenate/21
  String Constant12/1 -> String Concatenate/23
  String Constant13/1 -> String Concatenate/25
  String Constant14/1 -> String Concatenate/27
  String Constant15/1 -> String Concatenate/29
  String Constant16/1 -> String Concatenate/31
  String Constant17/1 -> String Concatenate/33
  String Constant18/1 -> String Concatenate/35
  " SRR_RelativeVelocity"/1 -> To String5/1
  To String5/1 -> String Concatenate/12
  " FLR_Range"/1 -> To String6/1
  To String6/1 -> String Concatenate/14
  " FLR_RelativeVelocity"/1 -> To String7/1
  To String7/1 -> String Concatenate/16
  FLR_Azimuth/1 -> To String8/1
  To String8/1 -> String Concatenate/18
  " FRR_Range"/1 -> To String9/1
  To String9/1 -> String Concatenate/20
  " FRR_RelativeVelocity"/1 -> To String10/1
  To String10/1 -> String Concatenate/22
  " FRR_Azimuth"/1 -> To String11/1
  To String11/1 -> String Concatenate/24
  " BRR_Range"/1 -> To String12/1
  To String12/1 -> String Concatenate/26
  " BRR_RelativeVelocity"/1 -> To String13/1
  To String13/1 -> String Concatenate/28
  " BRR_Azimuth"/1 -> To String14/1
  To String14/1 -> String Concatenate/30
  " BLR_Range"/1 -> To String15/1
  To String15/1 -> String Concatenate/32
  " BLR_RelativeVelocity"/1 -> To String16/1
  To String16/1 -> String Concatenate/34
  " BLR_Azimuth"/1 -> To String17/1
  To String17/1 -> String Concatenate/36
  String Constant19/1 -> String Concatenate/37
  To String18/1 -> String Concatenate/38
  Velocity/1 -> To String18/1
  String Constant5/1 -> String Concatenate/61
  To String19/1 -> String Concatenate/40
  laneMarkerX_D0/1 -> To String19/1
  String Constant20/1 -> String Concatenate/39
  String Constant21/1 -> String Concatenate/41
  To String20/1 -> String Concatenate/42
  laneMarkerY_D0/1 -> To String20/1
  String Constant22/1 -> String Concatenate/43
  To String21/1 -> String Concatenate/44
  laneMarkerX_D1/1 -> To String21/1
  String Constant23/1 -> String Concatenate/45
  To String22/1 -> String Concatenate/46
  laneMarkerY_D1/1 -> To String22/1
  String Constant24/1 -> String Concatenate/47
  To String23/1 -> String Concatenate/48
  worldrX_D0/1 -> To String23/1
  String Constant25/1 -> String Concatenate/49
  To String24/1 -> String Concatenate/50
  worldY_D0/1 -> To String24/1
  String Constant26/1 -> String Concatenate/51
  To String25/1 -> String Concatenate/52
  worldX_D1/1 -> To String25/1
  String Constant27/1 -> String Concatenate/53
  To String26/1 -> String Concatenate/54
  worldY_D1/1 -> To String26/1
  String Constant28/1 -> String Concatenate/55
  To String27/1 -> String Concatenate/56
  laneMarkerLeft_D1/1 -> To String27/1
  String Constant29/1 -> String Concatenate/57
  To String28/1 -> String Concatenate/58
  laneMarkerRight_D1/1 -> To String28/1
  String Constant30/1 -> String Concatenate/59
  To String29/1 -> String Concatenate/60
  roadID/1 -> To String29/1

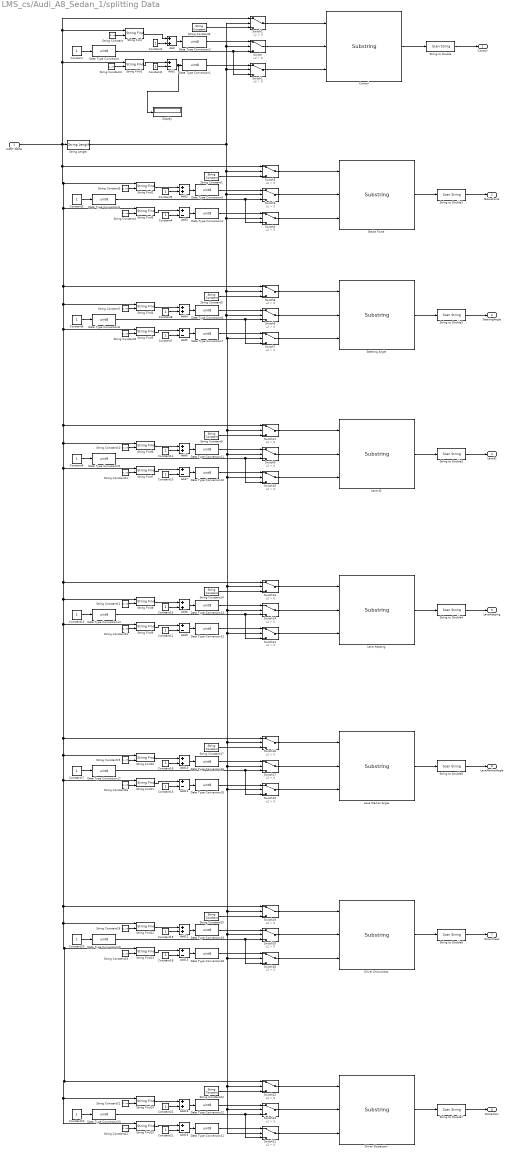
== system LMS_cs/Audi_A8_Sedan_1/splitting Data ==
  UART DATA : Inport
  Add{,2,4,6,8,10,12,14} (8 alike) : Sum
  Add{1,3,5,7,9,11,13,15} (8 alike) : Sum  Inputs=+-
  Brake Force : Substring
  Constant{,1..23} (24 alike) : Constant
  "Control " : Substring
  Data Type Conversion{,1..23} (24 alike) : DataTypeConversion  OutDataTypeStr=uint8  SaturateOnIntegerOverflow=off  RndMeth=Floor
  Display : Display
  Driver Distraction : Substring
  Driver Drowsiness : Substring
  Lane ID : Substring
  Lane Keeping : Substring
  Lane Marker Angle : Substring
  Steering Angle : Substring
  String Constant : StringConstant  String="\"*\""
  String Constant{1,5..6,9,14,17,20,23} (8 alike) : StringConstant  String="\"0\""
  String Constant10 : StringConstant  String="\"&\""
  String Constant11 : StringConstant  String="\"$\""
  String Constant12 : StringConstant  String="\"$\""
  String Constant13 : StringConstant  String="\"@\""
  String Constant15 : StringConstant  String="\"@\""
  String Constant16 : StringConstant  String="\"^\""
  String Constant18 : StringConstant  String="\"^\""
  String Constant19 : StringConstant  String="\"!\""
  String Constant2 : StringConstant  String="\";\""
  String Constant21 : StringConstant  String="\"!\""
  String Constant22 : StringConstant  String="\"#\""
  String Constant3 : StringConstant  String="\";\""
  String Constant4 : StringConstant  String="\"_\""
  String Constant7 : StringConstant  String="\"_\""
  String Constant8 : StringConstant  String="\"&\""
  String Find{,1..15} (16 alike) : StringFind
  String Length : StringLength
  String to Double{,1..7} (8 alike) : ScanString  Format="\"%lf\""
  Switch{,1..23} (24 alike) : Switch  Criteria=u2 > Threshold  SaturateOnIntegerOverflow=off  InputSameDT=off
  Control : Outport  VectorParamsAs1DForOutWhenUnconnected=off
  BrakeForce : Outport  Port=2  VectorParamsAs1DForOutWhenUnconnected=off
  SteeringAngle : Outport  Port=3  VectorParamsAs1DForOutWhenUnconnected=off
  LaneID : Outport  Port=4  VectorParamsAs1DForOutWhenUnconnected=off
  LaneKeeping : Outport  Port=5  VectorParamsAs1DForOutWhenUnconnected=off
  LaneMarkerAngle : Outport  Port=6  VectorParamsAs1DForOutWhenUnconnected=off
  Drowsiness : Outport  Port=7  VectorParamsAs1DForOutWhenUnconnected=off
  Distraction : Outport  Port=8  VectorParamsAs1DForOutWhenUnconnected=off
  wires:
  Constant/1 -> Data Type Conversion/1
  Switch2/1 -> "Control "/1
  Switch1/1 -> "Control "/3
  Switch/1 -> "Control "/2
  String Constant6/1 -> Switch2/3
  Data Type Conversion1/1 -> Switch1/1
  Data Type Conversion2/1 -> Switch/1
  Data Type Conversion/1 -> Switch/3, Switch1/3
  Data Type Conversion4/1 -> Switch4/1
  Switch4/1 -> Brake Force/3
  Switch5/1 -> Brake Force/1
  Data Type Conversion5/1 -> Switch3/1
  Data Type Conversion3/1 -> Switch3/3, Switch4/3
  Constant3/1 -> Data Type Conversion3/1
  String Constant1/1 -> Switch5/3
  Switch3/1 -> Brake Force/2
  "Control "/1 -> String to Double/1
  String to Double/1 -> Control/1
  Brake Force/1 -> String to Double1/1
  String to Double1/1 -> BrakeForce/1
  String Constant/1 -> String Find/2
  String Constant2/1 -> String Find1/2
  Constant1/1 -> Add/2
  Add/1 -> Data Type Conversion2/1
  String Find/1 -> Add/1
  Add1/1 -> Display/1, Data Type Conversion1/1
  Constant2/1 -> Add1/2
  String Find1/1 -> Add1/1
  Add2/1 -> Data Type Conversion5/1
  String Find2/1 -> Add2/1
  String Constant3/1 -> String Find2/2
  Constant5/1 -> Add2/2
  Add3/1 -> Data Type Conversion4/1
  Constant4/1 -> Add3/2
  String Find3/1 -> Add3/1
  String Constant4/1 -> String Find3/2
  Data Type Conversion8/1 -> Switch6/1
  String Constant8/1 -> String Find5/2
  String Constant5/1 -> Switch8/3
  Constant7/1 -> Add5/2
  Add5/1 -> Data Type Conversion7/1
  Constant8/1 -> Add4/2
  String Find4/1 -> Add4/1
  Add4/1 -> Data Type Conversion8/1
  Steering Angle/1 -> String to Double2/1
  String to Double2/1 -> SteeringAngle/1
  Constant6/1 -> Data Type Conversion6/1
  Switch7/1 -> Steering Angle/3
  Switch6/1 -> Steering Angle/2
  Data Type Conversion7/1 -> Switch7/1
  Data Type Conversion6/1 -> Switch6/3, Switch7/3
  String Constant7/1 -> String Find4/2
  String Find5/1 -> Add5/1
  Switch8/1 -> Steering Angle/1
  Data Type Conversion11/1 -> Switch9/1
  Add6/1 -> Data Type Conversion11/1
  String to Double3/1 -> LaneID/1
  Lane ID/1 -> String to Double3/1
  String Find6/1 -> Add6/1
  Switch10/1 -> Lane ID/3
  Constant9/1 -> Data Type Conversion9/1
  Data Type Conversion10/1 -> Switch10/1
  String Constant11/1 -> String Find7/2
  Constant10/1 -> Add7/2
  String Constant9/1 -> Switch11/3
  Constant11/1 -> Add6/2
  Switch9/1 -> Lane ID/2
  Switch11/1 -> Lane ID/1
  String Find7/1 -> Add7/1
  Data Type Conversion9/1 -> Switch9/3, Switch10/3
  Add7/1 -> Data Type Conversion10/1
  String Constant10/1 -> String Find6/2
  Constant13/1 -> Add8/2
  Switch13/1 -> Lane Keeping/1
  Add9/1 -> Data Type Conversion12/1
  String Constant12/1 -> String Find8/2
  String Constant13/1 -> String Find9/2
  Switch12/1 -> Lane Keeping/3
  String Constant14/1 -> Switch13/3
  Data Type Conversion14/1 -> Switch14/3, Switch12/3
  Data Type Conversion12/1 -> Switch12/1
  Switch14/1 -> Lane Keeping/2
  Constant14/1 -> Data Type Conversion14/1
  Data Type Conversion13/1 -> Switch14/1
  Constant12/1 -> Add9/2
  String Find8/1 -> Add8/1
  Add8/1 -> Data Type Conversion13/1
  String Find9/1 -> Add9/1
  Lane Keeping/1 -> String to Double4/1
  String to Double4/1 -> LaneKeeping/1
  String to Double5/1 -> LaneMarkerAngle/1
  String Find10/1 -> Add10/1
  Constant15/1 -> Add11/2
  Data Type Conversion16/1 -> Switch17/1
  Add10/1 -> Data Type Conversion16/1
  String Constant16/1 -> String Find11/2
  String Constant17/1 -> Switch16/3
  Lane Marker Angle/1 -> String to Double5/1
  Data Type Conversion15/1 -> Switch15/1
  Data Type Conversion17/1 -> Switch17/3, Switch15/3
  String Constant15/1 -> String Find10/2
  Add11/1 -> Data Type Conversion15/1
  Switch16/1 -> Lane Marker Angle/1
  Constant17/1 -> Data Type Conversion17/1
  String Find11/1 -> Add11/1
  Constant16/1 -> Add10/2
  Switch17/1 -> Lane Marker Angle/2
  Switch15/1 -> Lane Marker Angle/3
  Driver Drowsiness/1 -> String to Double6/1
  Switch18/1 -> Driver Drowsiness/3
  Switch19/1 -> Driver Drowsiness/1
  Constant20/1 -> Data Type Conversion20/1
  String Find13/1 -> Add13/1
  Add12/1 -> Data Type Conversion19/1
  Data Type Conversion18/1 -> Switch18/1
  String Constant18/1 -> String Find12/2
  Constant19/1 -> Add12/2
  Add13/1 -> Data Type Conversion18/1
  Data Type Conversion20/1 -> Switch20/3, Switch18/3
  String Find12/1 -> Add12/1
  String Constant20/1 -> Switch19/3
  String to Double6/1 -> Drowsiness/1
  Data Type Conversion19/1 -> Switch20/1
  String Constant19/1 -> String Find13/2
  Constant18/1 -> Add13/2
  Switch20/1 -> Driver Drowsiness/2
  Switch21/1 -> Driver Distraction/3
  Driver Distraction/1 -> String to Double7/1
  Data Type Conversion23/1 -> Switch23/3, Switch21/3
  Constant22/1 -> Add14/2
  Data Type Conversion21/1 -> Switch21/1
  String Constant21/1 -> String Find14/2
  Constant23/1 -> Data Type Conversion23/1
  Add15/1 -> Data Type Conversion21/1
  Add14/1 -> Data Type Conversion22/1
  Switch23/1 -> Driver Distraction/2
  Constant21/1 -> Add15/2
  Switch22/1 -> Driver Distraction/1
  String Constant22/1 -> String Find15/2
  UART DATA/1 -> String Find1/1, String Find/1, Switch2/1, String Length/1, String Find3/1, String Find6/1, String Find8/1, String Find10/1, String Find12/1, String Find14/1, String Find15/1, Switch22/1, String Find13/1, Switch19/1, String Find11/1, Switch16/1, String Find9/1, Switch13/1, String Find7/1, Switch11/1, String Find5/1, String Find4/1, Switch8/1, String Find2/1, Switch5/1
  String Constant23/1 -> Switch22/3
  String Find15/1 -> Add15/1
  String Length/1 -> Switch/2, Switch2/2, Switch1/2, Switch5/2, Switch3/2, Switch8/2, Switch21/2, Switch23/2, Switch22/2, Switch18/2, Switch20/2, Switch19/2, Switch15/2, Switch17/2, Switch16/2, Switch12/2, Switch14/2, Switch13/2, Switch10/2, Switch9/2, Switch11/2, Switch7/2, Switch6/2, Switch4/2
  Data Type Conversion22/1 -> Switch23/1
  String to Double7/1 -> Distraction/1
  String Find14/1 -> Add14/1

== system LMS_cs/BMW_X5_SUV_1/Dynamics_Simple_3D ==
  DeltaSteer_[deg] : Inport
  Throttle : Inport  Port=2
  Brake : Inport  Port=3
  Initial_Vx_[ms-1] : Inport  Port=4
  AutoManual_OnOff : Inport  Port=5
  Auto_GearShift : Inport  Port=6
  Manual_GearShift : Inport  Port=7
  TyreInfo_in : Inport  Port=8
  Bus Creator : BusCreator  Inputs=14
  Bus Selector : BusSelector  OutputSignals=z_wheelFL_[m],z_wheelFR_[m],z_wheelRL_[m],z_wheelRR_[m]
  Chassis : Subsystem
      mask Display: image(imread('Chassis.png'));
  Engine : Subsystem
      mask Display: image(imread('Engine.png'));
  Gain : Gain  Gain=3.6
  Gear: Auto Manual : Subsystem
  Mux : Mux  Inputs=3
  Radians to Degrees : simulink_extras/Transformations/Radians to Degrees
  Radians to Degrees1 : simulink_extras/Transformations/Radians to Degrees
  Selector : Selector  InputPortWidth=9  IndexOptions=Index vector (dialog)  Indices=7  OutputSizes=1
  Selector1 : Selector  InputPortWidth=9  IndexOptions=Index vector (dialog)  Indices=8  OutputSizes=1
  ShiftLogic : Subsystem
      mask Display: image(imread('Gearshift.png'));
  Transmission : Subsystem
      mask Display: image(imread('Transmission.png'));
  State : Outport
  Vx [m s-1] : Outport  Port=2
  Perf_Params : Outport  Port=3
  z_wheelFL_[m] : Outport  Port=4
  z_wheelFR_[m] : Outport  Port=5
  z_wheelRL_[m] : Outport  Port=6
  z_wheelRR_[m] : Outport  Port=7
  ContactParams : Outport  Port=8
  wires:
  [ax] -> Bus Creator/4  "Ax_[ms-2]"
  [vx] -> Gain/1
  Selector1/1 -> Radians to Degrees1/1
  Selector/1 -> Radians to Degrees/1
  [PD] -> Bus Creator/10  "PDrive_[kW]"
  Radians to Degrees1/1 -> Bus Creator/12  "Pitch_[deg]"
  Radians to Degrees/1 -> Bus Creator/11  "Roll_[deg]"
  [PE] -> Bus Creator/9  "PEngine_[kW]"
  Bus Creator/1 -> Perf_Params/1
  Engine/2(PEngine_[kW]) -> [PE]
  [brake] -> Bus Creator/8  "Brake_[bar]"
  [throttle] -> Bus Creator/7  "Throttle_[perc]"
  [auto_manual] -> Bus Creator/6  "Auto_Manual_[-]"
  [ay] -> Bus Creator/5  "Ay_[ms-2]"
  [gear] -> Bus Creator/3  "Gear_[-]"
  [RPM] -> Bus Creator/2  "NEngine_[rpm]"
  Gain/1 -> Bus Creator/1  "Vx_[kmh-1]"
  Transmission/1(ImpellerTorque_[Nm]) -> Engine/1(ImpellerTorque_[Nm])  "ImpellerTorque_[Nm]"
  Transmission/2(TransmissionTorque_[Nm]) -> Chassis/1(TransmissionTorque_[Nm])  "TransmissionTorque_[Nm]"
  ShiftLogic/1(GearNr) -> ShiftLogic/2(GearNr_[-]), Gear: Auto Manual/3(Auto_Gear)  "GearNr_[-]"
  Engine/1(nEngine_[rpm]) -> Transmission/1(nEngine_[rpm]), [RPM]  "nEngine_[rpm]"
  Chassis/1(State) -> Selector1/1, Selector/1, State/1, Mux/1
  DeltaSteer_[deg]/1 -> Chassis/3(DeltaSteer_[deg])
  Initial_Vx_[ms-1]/1 -> Chassis/4(Initial_Vx_[ms-1])
  Throttle/1 -> [throttle], ShiftLogic/1(Throttle_[%]), Engine/2(Throttle_[%])
  Auto_GearShift/1 -> ShiftLogic/3(Auto_GearShift)
  Chassis/7(TransmissionOut_[rpm]) -> Transmission/3(n_TransmissionOut_[rpm])  "n_driveline_[rpm]"
  Chassis/2(VehicleSpeed_[ms-1]) -> [vx], Vx [m s-1]/1, Mux/2  "vx_[ms-1]"
  AutoManual_OnOff/1 -> [auto_manual], Gear: Auto Manual/1(Auto_Manual)
  Manual_GearShift/1 -> Gear: Auto Manual/2(Manual_Gear)
  Gear: Auto Manual/1(Gear) -> [gear], Transmission/2(GearNr_[-])  "gear"
  [vx] -> ShiftLogic/4(VehSpeed_[ms-1])
  TyreInfo_in/1 -> Chassis/5(TyreInfo_in)
  Brake/1 -> Chassis/2(BrakePressure_[bar]), [brake]
  Chassis/6(PDrive_[kW]) -> [PD]
  Chassis/5(ay_[ms-2]) -> [ay]
  Chassis/4(ax_[ms-2]) -> [ax]
  Chassis/3(Vy_[ms-1]) -> [vy]
  [vx] -> Bus Creator/13  "vx_[ms-1]"
  [vy] -> Bus Creator/14  "vy_[ms-1]"
  Chassis/8(z_wheel_[m]) -> Bus Selector/1, Mux/3  "z_wheel_[m]"
  Bus Selector/1 -> z_wheelFL_[m]/1  "<z_wheelFL_[m]>"
  Bus Selector/2 -> z_wheelFR_[m]/1  "<z_wheelFR_[m]>"
  Bus Selector/3 -> z_wheelRL_[m]/1  "<z_wheelRL_[m]>"
  Bus Selector/4 -> z_wheelRR_[m]/1  "<z_wheelRR_[m]>"
  Mux/1 -> ContactParams/1

== system LMS_cs/BMW_X5_SUV_1/JointGroup_WheelDisplacement_V2R ==
  Velocity [m/s] : Inport  SampleTime=TimeStep
  Discrete-Time Integrator : DiscreteIntegrator  SampleTime=TimeStep  ICPrevOutput=DiscIntNeverNeededParam  ICPrevScaledInput=DiscIntNeverNeededParam
  omega=V/Rwheel : Gain  Gain=1/TireRadius
  Rotation [rad] : Outport
  wires:
  Discrete-Time Integrator/1 -> Rotation [rad]/1  "roty"
  omega=V/Rwheel/1 -> Discrete-Time Integrator/1  "rotational speed [rad/s]"
  Velocity [m/s]/1 -> omega=V/Rwheel/1
